simulink model "Test_per_emg"  (R2023b)
settings: Solver=VariableStepAuto  StartTime=0.0  StopTime=inf  RelTol=1e-3
undefined symbols (not defined in the file or in its folder): deg, m, s, t1, t2
libraries: qbmove_library x9, dspstat3 x2, CP_library x1, QB_pacer_lib x1
settings Model: Creator=ilari  LastModifiedBy=ilari

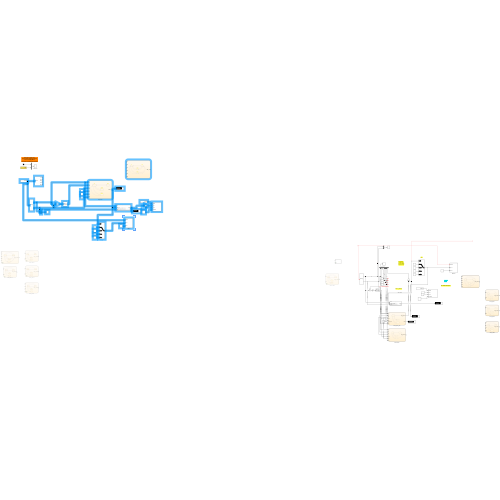
[thumbnail: Simulink's stored preview of the top-level diagram]
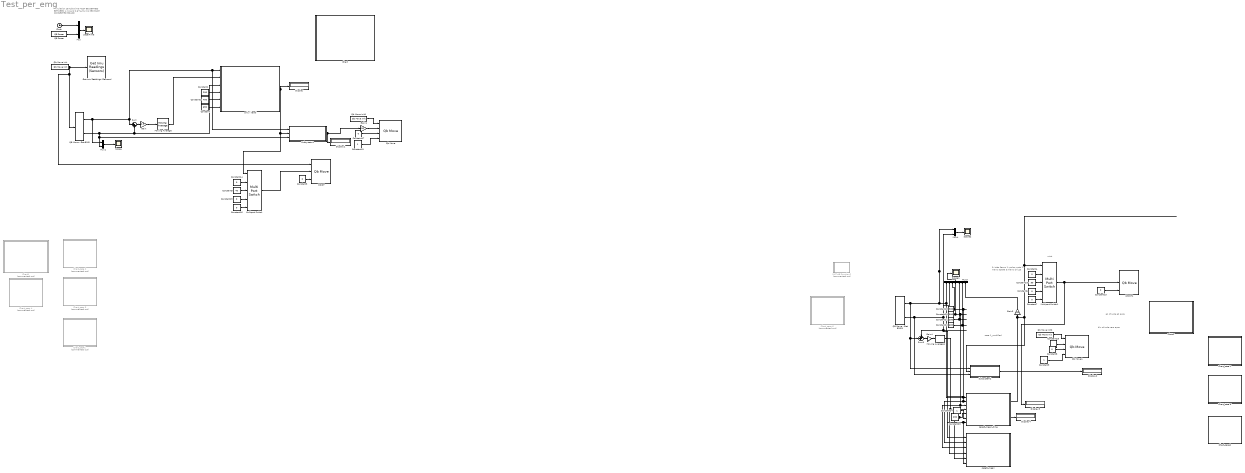
== system Test_per_emg ==
  note: Simulation sample time
      | MUST BE DEFINED BETWEEN
      | 1 ms and 0.6*N_IMU ms
      | PER EACH CONNECTED BOARD
  note: 0: tutto fermo
      | 1: polso ruota
      | 2: mano aperta
      | 3:mano chiusa
  note: wrist
  note: e1 chiude
      | e2 apre
  note: blu chiude nero apre
  note: case 1_modified
  Chart : Stateflow chart  TreatAsAtomicUnit=on
  Chart1 : Stateflow chart  Commented=on  TreatAsAtomicUnit=on
      settings: PortSchema="{\"entries\":[{\"content\":{\"sides\":[{\"content\":{\"connectorIds\":[\"In1\",\"In2\",\"In4\",\"In5\",\"In6\",\"In3\"]},\"type\":\"ConnectorPlacement.EquallySpacedRectSide\",\"uuid\":\"bb964aad-0f33-4b15-8f2f-07cc57dca142\"},{\"content\":{\"connectorIds\":[\"Out1\"],\"side\":\"RIGHT\"},\"type\":\"ConnectorPlacement.EquallySpacedRectSide\",\"uuid\":\"3d1bf315-7cf4-4964-aaea-501116c51cbb\"},{\"content\":{\"side\":\"TOP\"},\"type\":\"ConnectorPlacement.EquallySpacedRectSide\",\"uuid\":\"a0d71c19-2788-4f48-aff8-ceef882696bc\"}]},\"type\":\"ConnectorPlacement.EquallySpacedConnector\",\"uuid\":\"2eca7b29-df2d-4887-b2a9-df7a5d1fb129\"}],\"packageUris\":[\"http://schema.mathworks.com/mf0/Connector/R2020b\"],\"version\":\"1.0\"}"
  Chart2 : Stateflow chart  TreatAsAtomicUnit=on
      settings: PortSchema="{\"entries\":[{\"content\":{\"sides\":[{\"content\":{\"connectorIds\":[\"In1\",\"In2\",\"In4\",\"In5\",\"In6\",\"In3\"]},\"type\":\"ConnectorPlacement.EquallySpacedRectSide\",\"uuid\":\"bb964aad-0f33-4b15-8f2f-07cc57dca142\"},{\"content\":{\"connectorIds\":[\"Out1\"],\"side\":\"RIGHT\"},\"type\":\"ConnectorPlacement.EquallySpacedRectSide\",\"uuid\":\"3d1bf315-7cf4-4964-aaea-501116c51cbb\"},{\"content\":{\"side\":\"TOP\"},\"type\":\"ConnectorPlacement.EquallySpacedRectSide\",\"uuid\":\"a0d71c19-2788-4f48-aff8-ceef882696bc\"}]},\"type\":\"ConnectorPlacement.EquallySpacedConnector\",\"uuid\":\"2eca7b29-df2d-4887-b2a9-df7a5d1fb129\"}],\"packageUris\":[\"http://schema.mathworks.com/mf0/Connector/R2020b\"],\"version\":\"1.0\"}"
  Chart_case 1 : Stateflow chart  TreatAsAtomicUnit=on
  Chart_case 2 : Stateflow chart  Commented=on  TreatAsAtomicUnit=on
  Chart_case 3 : Stateflow chart  Commented=on  TreatAsAtomicUnit=on
  Chart_case 4 : Stateflow chart  Commented=on  TreatAsAtomicUnit=on
  Chart_case 5 : Stateflow chart  TreatAsAtomicUnit=on
  Chart_case 6 : Stateflow chart  Commented=on  TreatAsAtomicUnit=on
  Chart_case1 : Stateflow chart  Commented=on  TreatAsAtomicUnit=on
  Chart_case2 : Stateflow chart  TreatAsAtomicUnit=on
  Clock : Clock
  Constant : Constant  Value=650
  Constant1 : Constant  Value=200
  Constant10 : Constant  Value=50
  Constant{3..4,6..8,13..17} (10 alike) : Constant  Value=0
  Constant18 : Constant  Value=300
  Constant19 : Constant
  Constant2 : Constant  Value=400
  Constant20 : Constant  Value=500
  Constant21 : Constant  Value=200
  Constant22 : Constant  Value=600
  Constant23 : Constant  Value=230
  Constant24 : Constant
  Constant25 : Constant  Value=10000
  Constant5 : Constant  Value=40
  Constant9 : Constant
  Display{,1..4} (5 alike) : Display
  Gain : Gain  Gain=0.5
  Gain1 : Gain  Gain=50
  Gain3 : Gain  Gain=100
  Gain4 : Gain  Gain=0.5
  Get Imu Readings (Sensors) : CP_library/Get Imu Readings (Sensors)  ID=2  N_IMU=1  DAISY_CHAINING=off  ACC_UNITY=m/(s^2)  GYRO_UNITY=deg/s  MAG_UNITY=uT
      settings: SourceProductName=Centro Piaggio Library
  MATLAB Function5 : MATLAB Function  Commented=on  TreatAsAtomicUnit=on
  Moving Average : dspstat3/Moving Average  Method=Sliding window  ForgettingFactorPort=off  SpecifyWindowLength=on  WindowLength=4  OverlapLength=3  AllowArbitraryInputLength=off  ForgettingFactor=0.9  SimulateUsing=Code generation
  Moving Average1 : dspstat3/Moving Average  Method=Sliding window  ForgettingFactorPort=off  SpecifyWindowLength=on  WindowLength=4  OverlapLength=3  AllowArbitraryInputLength=off  ForgettingFactor=0.9  SimulateUsing=Code generation
  Multiport Switch : MultiPortSwitch  DataPortOrder=Zero-based contiguous  Inputs=4  zeroidx=on  SaturateOnIntegerOverflow=off  InputSameDT=off
  Multiport Switch1 : MultiPortSwitch  DataPortOrder=Zero-based contiguous  Inputs=4  zeroidx=on  SaturateOnIntegerOverflow=off  InputSameDT=off
  Mux : Mux  Inputs=2
  Mux1 : Mux  Inputs=2
  Mux3 : Mux  Inputs=7
  Mux4 : Mux  Inputs=2
  QB Move - Get EMG : qbmove_library/QB Move - Get EMG  ID=2  DAISY_CHAINING=off
      settings: SourceProductName=Qb Move Library
  QB Move - Get EMG1 : qbmove_library/QB Move - Get EMG  ID=2  DAISY_CHAINING=off
      settings: SourceProductName=Qb Move Library
  QB Pacer : QB_pacer_lib/QB Pacer  simTimePerRealTime=1
      settings: SourceProductName=QB Pacer
  Qb Move : qbmove_library/Qb Move  ID=1  ACTIVE_COMM_DIRECTIONS=Tx  CONTROL_MODE=Prime Movers Positions  DAISY_CHAINING=off  MAX_ANG=0  SW_LIMIT=inf  OFFSET=0  ACTIVATE=off  WDT=0.0  UNIT=TICK
      settings: LibrarySourceBlock=qbmove_library/qbmove  SourceProductName=Qb Move Library
  Qb Move Init : qbmove_library/Qb Move Init  NUMBER_OF_COM='COM9'  BAUD_RATE_COM=2000000
      settings: SourceProductName=Qb Move Library
  Qb Move Init1 : qbmove_library/Qb Move Init  NUMBER_OF_COM='COM7'  BAUD_RATE_COM=2000000
      settings: SourceProductName=Qb Move Library
  Qb Move Init2 : qbmove_library/Qb Move Init  NUMBER_OF_COM='COM7'  BAUD_RATE_COM=2000000
      settings: SourceProductName=Qb Move Library
  Qb Move1 : qbmove_library/Qb Move  ID=1  ACTIVE_COMM_DIRECTIONS=Tx  CONTROL_MODE=Prime Movers Positions  DAISY_CHAINING=off  MAX_ANG=0  SW_LIMIT=inf  OFFSET=0  ACTIVATE=off  WDT=0.0  UNIT=TICK
      settings: LibrarySourceBlock=qbmove_library/qbmove  SourceProductName=Qb Move Library
  Scope : Scope
  Scope1 : Scope
  Scope2 : Scope
  Subsystem1 : Subsystem
  Subsystem2 : Subsystem
  Sum : Sum  Inputs=|++
  Sum3 : Sum  Inputs=++|
  WRIST : qbmove_library/Qb Move  ID=2  ACTIVE_COMM_DIRECTIONS=Tx  CONTROL_MODE=Prime Movers Positions  DAISY_CHAINING=off  MAX_ANG=0  SW_LIMIT=inf  OFFSET=0  ACTIVATE=on  WDT=0.0  UNIT=TICK
      settings: SourceProductName=Qb Move Library
  WRIST1 : qbmove_library/Qb Move  ID=2  ACTIVE_COMM_DIRECTIONS=Tx  CONTROL_MODE=Prime Movers Positions  DAISY_CHAINING=off  MAX_ANG=0  SW_LIMIT=inf  OFFSET=0  ACTIVATE=on  WDT=0.0  UNIT=TICK
      settings: SourceProductName=Qb Move Library
  case5_mean : Stateflow chart  TreatAsAtomicUnit=on
      settings: PortSchema="{\"entries\":[{\"content\":{\"sides\":[{\"content\":{\"connectorIds\":[\"In1\",\"In2\",\"In4\",\"In6\",\"In5\",\"In3\"]},\"type\":\"ConnectorPlacement.EquallySpacedRectSide\",\"uuid\":\"bb964aad-0f33-4b15-8f2f-07cc57dca142\"},{\"content\":{\"connectorIds\":[\"Out1\"],\"side\":\"RIGHT\"},\"type\":\"ConnectorPlacement.EquallySpacedRectSide\",\"uuid\":\"3d1bf315-7cf4-4964-aaea-501116c51cbb\"},{\"content\":{\"side\":\"TOP\"},\"type\":\"ConnectorPlacement.EquallySpacedRectSide\",\"uuid\":\"a0d71c19-2788-4f48-aff8-ceef882696bc\"}]},\"type\":\"ConnectorPlacement.EquallySpacedConnector\",\"uuid\":\"2eca7b29-df2d-4887-b2a9-df7a5d1fb129\"}],\"packageUris\":[\"http://schema.mathworks.com/mf0/Connector/R2020b\"],\"version\":\"1.0\"}"
  case5_mean_time : Stateflow chart  TreatAsAtomicUnit=on
      settings: PortSchema="{\"entries\":[{\"content\":{\"sides\":[{\"content\":{\"connectorIds\":[\"In1\",\"In2\",\"In4\",\"In5\",\"In6\",\"In7\",\"In3\"]},\"type\":\"ConnectorPlacement.EquallySpacedRectSide\",\"uuid\":\"bb964aad-0f33-4b15-8f2f-07cc57dca142\"},{\"content\":{\"connectorIds\":[\"Out1\",\"Out2\"],\"side\":\"RIGHT\"},\"type\":\"ConnectorPlacement.EquallySpacedRectSide\",\"uuid\":\"3d1bf315-7cf4-4964-aaea-501116c51cbb\"},{\"content\":{\"side\":\"TOP\"},\"type\":\"ConnectorPlacement.EquallySpacedRectSide\",\"uuid\":\"a0d71c19-2788-4f48-aff8-ceef882696bc\"}]},\"type\":\"ConnectorPlacement.EquallySpacedConnector\",\"uuid\":\"2eca7b29-df2d-4887-b2a9-df7a5d1fb129\"}],\"packageUris\":[\"http://schema.mathworks.com/mf0/Connector/R2020b\"],\"version\":\"1.0\"}"
  only I level : Stateflow chart  TreatAsAtomicUnit=on
  pacerTime : Scope
  wires:
  Mux/1 -> pacerTime/1
  Clock/1 -> Mux/1
  QB Pacer/1 -> Mux/2
  Qb Move Init/1 -> WRIST/1, QB Move - Get EMG/1, Get Imu Readings (Sensors)/1
  QB Move - Get EMG/1 -> Mux1/1, Sum/1, only I level/1(e1), Subsystem1/1(e1)  "e1"
  QB Move - Get EMG/2 -> Mux1/2, Subsystem1/3(e2), only I level/3(e2), Sum/2  "e2"
  Sum/1 -> Gain/1
  Gain/1 -> Moving Average/1
  only I level/1(state_var) -> Multiport Switch/1, Subsystem1/2(In2), Display/1
  Constant/1 -> only I level/6(th2)
  Constant1/1 -> only I level/4(tm)
  Moving Average/1 -> only I level/2(em)
  Mux1/1 -> Scope/1
  Constant2/1 -> only I level/5(th1)
  Constant17/1 -> Qb Move/3
  Constant19/1 -> Qb Move/4
  Qb Move Init1/1 -> Qb Move/1
  Constant3/1 -> WRIST/3
  Multiport Switch/1 -> WRIST/2
  Constant16/1 -> Multiport Switch/5
  Constant14/1 -> Multiport Switch/2
  Constant15/1 -> Multiport Switch/4
  Constant5/1 -> Multiport Switch/3
  Subsystem1/1(Out1) -> Gain1/1, Display1/1
  Gain1/1 -> Qb Move/2
  Gain3/1 -> Mux3/7
  Constant24/1 -> case5_mean_time/7(time_min)
  Constant9/1 -> Qb Move1/4
  Gain4/1 -> Moving Average1/1
  Multiport Switch1/1 -> WRIST1/2, Display3/1
  case5_mean_time/2(time) -> Display4/1
  Constant6/1 -> Multiport Switch1/4
  Constant23/1 -> case5_mean_time/6(tm), case5_mean/5(tm)
  Qb Move Init2/1 -> Qb Move1/1
  Constant21/1 -> Mux3/5  "t3"
  Subsystem2/1(Out1) -> Display2/1
  Constant18/1 -> case5_mean/2(t1), case5_mean_time/2(t1), Mux3/3  "t1"
  Constant22/1 -> Mux3/6  "t4"
  Constant13/1 -> WRIST1/3
  Sum3/1 -> Gain4/1
  Mux3/1 -> Scope1/1
  Constant7/1 -> Multiport Switch1/5
  Constant4/1 -> Multiport Switch1/2
  Constant8/1 -> Qb Move1/3
  QB Move - Get EMG1/1 -> Mux4/1, Mux3/1, case5_mean/1(e1), case5_mean_time/1(e1), Sum3/2, Subsystem2/1(e1)  "e1"
  QB Move - Get EMG1/2 -> case5_mean/3(e2), case5_mean_time/3(e2), Sum3/1, Mux3/2, Mux4/2, Subsystem2/3(e2)  "e2"
  case5_mean_time/1(emg_control) -> Subsystem2/2(In2), Multiport Switch1/1, Gain3/1  "emg_control"
  Constant20/1 -> case5_mean_time/4(t2), case5_mean/4(t2), Mux3/4  "t2"
  Mux4/1 -> Scope2/1
  Constant10/1 -> Multiport Switch1/3
  Moving Average1/1 -> case5_mean_time/5(em), case5_mean/6(em)  "em"
  ? -> WRIST1/1
  ? -> QB Move - Get EMG1/1
  Constant25/1 -> Qb Move1/2

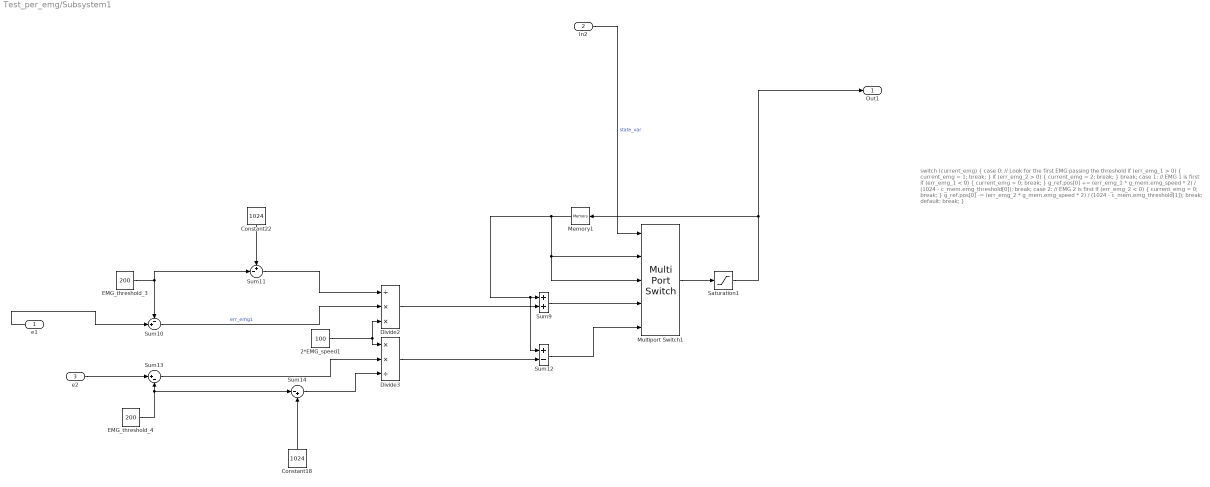
== system Test_per_emg/Subsystem1 ==
  note: switch (current_emg) {
      | case 0:
      | // Look for the first EMG passing the threshold
      | if (err_emg_1 > 0) {
      | current_emg = 1;
      | break;
      | }
      | if (err_emg_2 > 0) {
      | current_emg = 2;
      | break;
      | }
      | break;
      |
      | case 1:
      | // EMG 1 is first
      | if (err_emg_1 < 0) {
      | current_emg = 0;
      | break;
      | }
      | g_ref.pos[0] += (err_emg_1 * g_mem.emg_speed * 2) / (1024 - c_mem.emg_threshold[0]);
      | break;
      |
      | case 2:
      | // EMG 2 is first
      | if (err_emg_2 < 0) {
      | current_emg = 0;
      | break;
      | }
      | g_ref.pos[0] -= (err_emg_2 * g_mem.emg_speed * 2) / (1024 - c_mem.emg_threshold[1]);
      | break;
      |
      | default:
      | break;
      | }
  e1 : Inport
  In2 : Inport  Port=2
  e2 : Inport  Port=3
  2*EMG_speed1 : Constant  Value=100
  Constant18 : Constant  Value=1024
  Constant22 : Constant  Value=1024
  Divide2 : Product  Inputs=/**
  Divide3 : Product  Inputs=**/
  EMG_threshold_3 : Constant  Value=200
  EMG_threshold_4 : Constant  Value=200
  Memory1 : Memory
  Multiport Switch1 : MultiPortSwitch  DataPortOrder=Zero-based contiguous  Inputs=4  zeroidx=on  SaturateOnIntegerOverflow=off  InputSameDT=off
  Saturation1 : Saturate  UpperLimit=17500  LowerLimit=0
  Sum10 : Sum  Inputs=-+|
  Sum11 : Sum  Inputs=+-|
  Sum12 : Sum  Inputs=+-
  Sum13 : Sum  Inputs=|+-
  Sum14 : Sum  Inputs=|-+
  Sum9 : Sum
  Out1 : Outport
  wires:
  Multiport Switch1/1 -> Saturation1/1
  Memory1/1 -> Multiport Switch1/2, Multiport Switch1/3, Sum12/1, Sum9/1
  e1/1 -> Sum10/2
  Sum11/1 -> Divide2/1
  Sum9/1 -> Multiport Switch1/4
  Saturation1/1 -> Out1/1, Memory1/1
  Divide2/1 -> Sum9/2
  Divide3/1 -> Sum12/2
  Sum14/1 -> Divide3/3
  EMG_threshold_3/1 -> Sum11/2, Sum10/1
  EMG_threshold_4/1 -> Sum14/1, Sum13/2
  Constant18/1 -> Sum14/2
  2*EMG_speed1/1 -> Divide3/1, Divide2/3
  Sum13/1 -> Divide3/2
  e2/1 -> Sum13/1
  Sum12/1 -> Multiport Switch1/5
  Sum10/1 -> Divide2/2  "err_emg1"
  Constant22/1 -> Sum11/1
  In2/1 -> Multiport Switch1/1  "state_var"

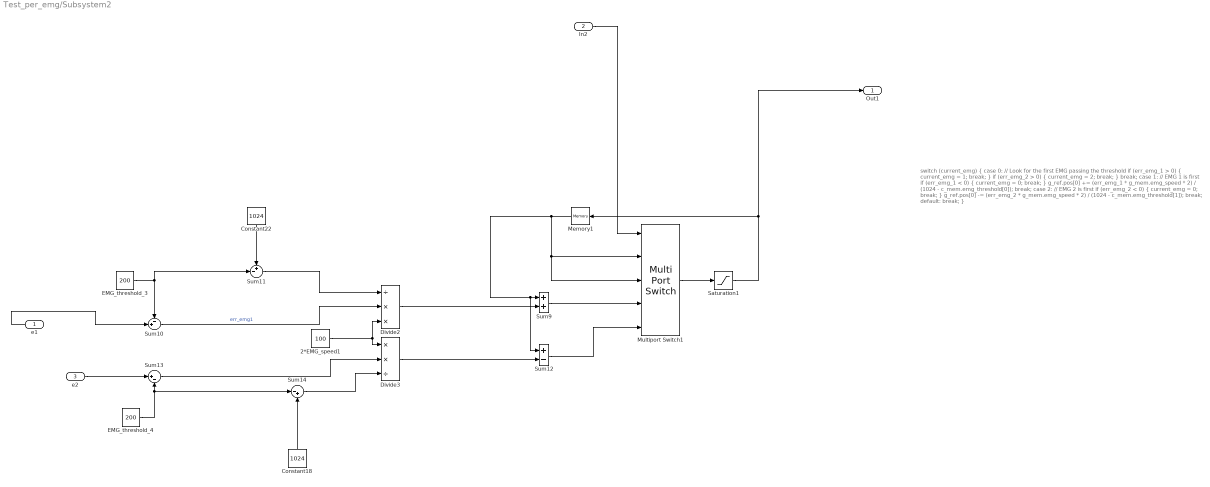
== system Test_per_emg/Subsystem2 ==
  note: switch (current_emg) {
      | case 0:
      | // Look for the first EMG passing the threshold
      | if (err_emg_1 > 0) {
      | current_emg = 1;
      | break;
      | }
      | if (err_emg_2 > 0) {
      | current_emg = 2;
      | break;
      | }
      | break;
      |
      | case 1:
      | // EMG 1 is first
      | if (err_emg_1 < 0) {
      | current_emg = 0;
      | break;
      | }
      | g_ref.pos[0] += (err_emg_1 * g_mem.emg_speed * 2) / (1024 - c_mem.emg_threshold[0]);
      | break;
      |
      | case 2:
      | // EMG 2 is first
      | if (err_emg_2 < 0) {
      | current_emg = 0;
      | break;
      | }
      | g_ref.pos[0] -= (err_emg_2 * g_mem.emg_speed * 2) / (1024 - c_mem.emg_threshold[1]);
      | break;
      |
      | default:
      | break;
      | }
  e1 : Inport
  In2 : Inport  Port=2
  e2 : Inport  Port=3
  2*EMG_speed1 : Constant  Value=100
  Constant18 : Constant  Value=1024
  Constant22 : Constant  Value=1024
  Divide2 : Product  Inputs=/**
  Divide3 : Product  Inputs=**/
  EMG_threshold_3 : Constant  Value=200
  EMG_threshold_4 : Constant  Value=200
  Memory1 : Memory
  Multiport Switch1 : MultiPortSwitch  DataPortOrder=Zero-based contiguous  Inputs=4  zeroidx=on  SaturateOnIntegerOverflow=off  InputSameDT=off
  Saturation1 : Saturate  UpperLimit=17500  LowerLimit=0
  Sum10 : Sum  Inputs=-+|
  Sum11 : Sum  Inputs=+-|
  Sum12 : Sum  Inputs=+-
  Sum13 : Sum  Inputs=|+-
  Sum14 : Sum  Inputs=|-+
  Sum9 : Sum
  Out1 : Outport
  wires:
  Multiport Switch1/1 -> Saturation1/1
  Memory1/1 -> Multiport Switch1/2, Multiport Switch1/3, Sum12/1, Sum9/1
  e1/1 -> Sum10/2
  Sum11/1 -> Divide2/1
  Sum9/1 -> Multiport Switch1/4
  Saturation1/1 -> Out1/1, Memory1/1
  Divide2/1 -> Sum9/2
  Divide3/1 -> Sum12/2
  Sum14/1 -> Divide3/3
  EMG_threshold_3/1 -> Sum11/2, Sum10/1
  EMG_threshold_4/1 -> Sum14/1, Sum13/2
  Constant18/1 -> Sum14/2
  2*EMG_speed1/1 -> Divide3/1, Divide2/3
  Sum13/1 -> Divide3/2
  e2/1 -> Sum13/1
  Sum12/1 -> Multiport Switch1/5
  Sum10/1 -> Divide2/2  "err_emg1"
  Constant22/1 -> Sum11/1
  In2/1 -> Multiport Switch1/1

== stateflow chart Test_per_emg/Chart_case 1 ==
  state State0
    entry: emg_control =0;
  state State1
    entry: emg_control=1;
  state State2
    entry: emg_control =2;
  state State3
    entry: emg_control=3;
  State1 -> State0 : [e2>t1 & e2<t2]
  (default) -> State0
  State0 -> State1 [order 2] : [e1>t1 & e1<t2]
  State0 -> State3 [order 3] : [e2>t2]
  State3 -> State0 : [e2<t2]
  State0 -> State2 [order 1] : [e1>t2]
  State2 -> State0 : [e1<t2]
  data: e1 input; e2 input; emg_control output; t2 parameter; t1 parameter

== stateflow chart Test_per_emg/Chart_case 5 ==
  state State0
    entry: emg_control =0;
  state State1
    entry: emg_control=1;
  state State2
    entry: emg_control =2;
  state State3
    entry: emg_control=3;
  State1 -> State0 : [e1>t1 & e1<t2]
  (default) -> State0
  State0 -> State1 [order 2] : [e2>t1 & e2<t2]
  State0 -> State3 [order 3] : [e2>t2]
  State3 -> State0 : [e2<t2]
  State0 -> State2 [order 1] : [e1>t2]
  State2 -> State0 : [e1<t2]
  data: e1 input; e2 input; emg_control output; t2 parameter; t1 parameter

== stateflow chart Test_per_emg/Chart_case 4 ==
  state State0
    entry: emg_control =0;
  state State1
    entry: emg_control=1;
  state State2
    entry: emg_control =2;
  state State3
    entry: emg_control=3;
  State1 -> State0 [order 2] : [e2>t1 & e2<t2]
  State1 -> State0 [order 1] : [e1>t1 & e1<t2]
  (default) -> State0
  State0 -> State1 [order 2] : [e1>t1 & e1<t2]
  State0 -> State1 [order 4] : [e2>t1 & e2<t2]
  State0 -> State3 [order 3] : [e2>t2]
  State3 -> State0 : [e2<t2]
  State0 -> State2 [order 1] : [e1>t2]
  State2 -> State0 : [e1<t2]
  data: e1 input; e2 input; emg_control output; t2 parameter; t1 parameter

== stateflow chart Test_per_emg/Chart1 ==
  state State0
    entry: emg_control =0;
  state State1
    entry: emg_control=1;
  state State2
    entry: emg_control =2;
  state State3
    entry: emg_control=3;
  State1 -> State0 [order 2] : [e1<t3]
  State1 -> State0 [order 1] : [e1<t3]
  (default) -> State0
  State0 -> State1 [order 2] : [e1>t1 & e1<t2]
  State0 -> State1 [order 4] : [e2>t1 & e2<t2]
  State1 -> State2 [order 4] : [e1>t4]
  State2 -> State1 [order 2] : [e1>t1 & e1<t2]
  State1 -> State3 [order 3] : [e2>t4]
  State3 -> State1 [order 2] : [e2>t1 & e2<t2]
  State0 -> State3 [order 3] : [e2>t2]
  State3 -> State0 [order 1] : [e2<t1]
  State0 -> State2 [order 1] : [e1>t2]
  State2 -> State0 [order 1] : [e1<t1]
  data: e1 input; t1 input; e2 input; t2 input; t3 input; t4 input; emg_control output

== stateflow chart Test_per_emg/Chart_case 2 ==
  state State0
    entry: emg_control =0;
  state State1
    entry: emg_control=1;
  state State2
    entry: emg_control =2;
  state State3
    entry: emg_control=3;
  State1 -> State0 : [e2>t1 & e2<t2]
  (default) -> State0
  State0 -> State1 [order 2] : [e1>t1 & e1<t2]
  State0 -> State3 [order 3] : [e2>t2]
  State3 -> State0 : [e2<t2]
  State0 -> State2 [order 1] : [e1>t2]
  State2 -> State0 : [e1<t2]
  data: e1 input; e2 input; emg_control output; t2 parameter; t1 parameter

== stateflow chart Test_per_emg/Chart_case 3 ==
  state State0
    entry: emg_control =0;
  state State1
    entry: emg_control=1;
  state State2
    entry: emg_control =2;
  state State3
    entry: emg_control=3;
  State1 -> State0 : [e1>t1 & e1<t2]
  (default) -> State0
  State0 -> State1 [order 2] : [e2>t1 & e2<t2]
  State0 -> State3 [order 3] : [e2>t2]
  State3 -> State0 : [e2<t2]
  State0 -> State2 [order 1] : [e1>t2]
  State2 -> State0 : [e1<t2]
  data: e1 input; e2 input; emg_control output; t2 parameter; t1 parameter

== stateflow chart Test_per_emg/Chart_case1 ==
  state State0
    entry: emg_control =0;
  state State1
    entry: emg_control=1;
  state State2
    entry: emg_control =2;
  state State3
    entry: emg_control=3;
  State1 -> State0 [order 2] : [e2>t2]
  State1 -> State0 [order 1] : [e1>t2]
  (default) -> State0
  State0 -> State1 [order 2] : [e1>t1 & e1<t2]
  State0 -> State1 [order 4] : [e2>t1 & e2<t2]
  State0 -> State3 [order 3] : [e2>t2]
  State3 -> State0 : [e2<t2]
  State0 -> State2 [order 1] : [e1>t2]
  State2 -> State0 : [e1<t2]
  data: e1 input; t1 input; t2 input; e2 input; emg_control output

== stateflow chart Test_per_emg/Chart_case 6 ==
  state State0
    entry: emg_control =0;
  state State1
    entry: emg_control=1;
  state State2
    entry: emg_control =2;
  state State3
    entry: emg_control=3;
  State1 -> State0 [order 2] : [e2>t1 & e2<t2]
  State1 -> State0 [order 1] : [e1>t1 & e1<t2]
  (default) -> State0
  State0 -> State1 [order 2] : [e1>t1 & e1<t2]
  State0 -> State1 [order 4] : [e2>t1 & e2<t2]
  State0 -> State3 [order 3] : [e2>t2]
  State3 -> State0 : [e2<t2]
  State0 -> State2 [order 1] : [e1>t2]
  State2 -> State0 : [e1<t2]
  data: e1 input; e2 input; emg_control output; t2 parameter; t1 parameter

== stateflow chart Test_per_emg/Chart_case2 ==
  state State0
    entry: emg_control =0;
  state State1
    entry: emg_control=1;
  state State2
    entry: emg_control =2;
  state State3
    entry: emg_control=3;
  State1 -> State0 [order 2] : [e2>t2]
  State1 -> State0 [order 1] : [e1>t2]
  (default) -> State0
  State0 -> State1 [order 2] : [e1>t1 & e1<t2]
  State0 -> State1 [order 4] : [e2>t1 & e2<t2]
  State0 -> State3 [order 3] : [e2>t2]
  State3 -> State0 : [e2<t2]
  State0 -> State2 [order 1] : [e1>t2]
  State2 -> State0 : [e1<t2]
  data: e1 input; t1 input; t2 input; e2 input; emg_control output

== matlab function Test_per_emg/MATLAB Function5 ==
  data: e1 input; e2 input
function  plot_emg(e1,e2)
figure(1)
hold on

yline(ax, 0.5, '--k', 'Linea di riferimento 1');
yline(ax, -0.5, '--k', 'Linea di riferimento 2');
plot (e1)
end

% persistent fig ax label_handle time
% 
% % Inizializza il grafico al primo ciclo
% if isempty(fig)
%     fig = figure;
%     ax = axes('Parent', fig);
%     hold(ax, 'on');
%     plot(ax, NaN, NaN, 'b', 'DisplayName', 'e1');
%     plot(ax, NaN, NaN, 'r', 'DisplayName', 'e2');
% 
%     % Aggiungi linee orizzontali di riferimento
%     yline(ax, 0.5, '--k', 'Linea di riferimento 1');
%     yline(ax, -0.5, '--k', 'Linea di riferimento 2');
% 
%     % Configura il grafico
%     xlabel(ax, 'Tempo (s)');
%     ylabel(ax, 'Valore');
%     title(ax, 'Grafico con etichetta dinamica e linee di riferimento');
%     legend(ax, 'show');
% 
%     time = 0;  % inizializza il tempo
% end
% 
% % Aggiorna il tempo a ogni chiamata (in Simulink questo viene aggiornato a ogni step)
% time = time + 0.1; % aggiorna il tempo, usando il passo di simulazione desiderato
% 
% % Plotta i dati aggiornati
% plot(ax, time, e1, 'bo');
% plot(ax, time, e2, 'ro');
% 
% % Crea o aggiorna l'etichetta dinamica
% if e1 > 0.7 && e2 > 0.7
%     label_text = 'Entrambi i segnali sopra la soglia 1';
% elseif e1 < -0.7 && e2 < -0.7
%     label_text = 'Entrambi i segnali sotto la soglia 2';
% else
%     label_text = 'Condizione neutrale';
% end
% 
% % Aggiorna o crea l'oggetto del testo
% if isempty(label_handle)
%     label_handle = text(time, max(e1, e2) + 0.1, label_text, ...
%         'FontSize', 10, 'FontWeight', 'bold', 'Color', 'm', 'Parent', ax);
% else
%     set(label_handle, 'Position', [time, max(e1, e2) + 0.1, 0], 'String', label_text);
% end
% 
% % Aggiorna gli assi per mantenere visibile l'ultimo valore
% xlim(ax, [max(0, time - 10), time + 1]); % visualizza solo gli ultimi 10 secondi
% 
% end

== stateflow chart Test_per_emg/case5_mean ==
  state State0
    entry: emg_control =0;
  state State1
    entry: emg_control=1;
  state State2
    entry: emg_control =2;
  state State3
    entry: emg_control=3;
  (default) -> State0
  State0 -> State1 [order 1] : [em>tm & e1<t2 & e2<t2]
  State1 -> State3 [order 2] : [em>tm & e1<t2 & e2>t2]
  State1 -> State0 [order 1] : [em<tm ]
  State1 -> State2 [order 3] : [em>tm & e1>t2 & e2<tm]
  State0 -> State3 [order 3] : [em>tm & e1<t2 & e2>t2]
  State3 -> State0 : [e2<t2]
  State2 -> State0 : [e1<t2 ]
  State0 -> State2 [order 2] : [em>tm & e1>t2 & e2<t2]
  data: e1 input; t1 input; e2 input; t2 input; tm input; emg_control output; em input

== stateflow chart Test_per_emg/case5_mean_time ==
  state State0
    entry: emg_control =0;
    entry: time =0;
    during: time = time +1;
    exit: time=0;
  state State1
    entry: emg_control=1;
  state State2
    entry: emg_control =2;
  state State3
    entry: emg_control=3;
  (default) -> State0
  State0 -> State1 [order 1] : [em>tm & e1<t2 & e2<t2 & time>time_min]
  State1 -> State0 : [em<tm & time>time_min]
  State0 -> State3 [order 3] : [em>tm & e1<t2 & e2>t1 & time>time_min]
  State3 -> State0 : [e2<t2 & time>time_min]
  State2 -> State0 : [e1<t2 & time>time_min]
  State0 -> State2 [order 2] : [em>tm & e1>t2 & e2<t2 & time>time_min]
  data: e1 input; t1 input; e2 input; t2 input; emg_control output; em input; tm input; time_min input; time output

== stateflow chart Test_per_emg/only I level ==
  note: rest
  note: polso on
  state state0
    entry: state_var = 0;
  state state1
    entry: state_var=1;
  note: mano chiusa
  state state2
    entry: state_var=2;
  note: mano aperta
  state state3
    entry: state_var=3;
  (default) -> state0
  state0 -> state1 [order 1] : [em>tm & e1<th1 & e2<th2]
  state1 -> state0 : [em<tm]
  state3 -> state0 : [em<tm & e2<th2]
  state0 -> state3 [order 3] : [em>tm & e2>th2]
  state0 -> state2 [order 2] : [em<tm & e1>th1]
  state2 -> state0 : [em<tm & e1<th1]
  data: e1 input; em input size=1; e2 input; tm input; th1 input; state_var output; th2 input

== stateflow chart Test_per_emg/Chart2 ==
  state State0
    entry: emg_control =0;
  state State1
    entry: emg_control=1;
  state State2
    entry: emg_control =2;
  state State3
    entry: emg_control=3;
  State1 -> State0 [order 2] : [e1<t3]
  State1 -> State0 [order 1] : [e1<t3]
  (default) -> State0
  State0 -> State1 [order 2] : [e1>t1 & e1<t2]
  State0 -> State1 [order 4] : [e2>t1 & e2<t2]
  State1 -> State2 [order 4] : [e1>t4]
  State2 -> State1 [order 2] : [e1>t1 & e1<t2]
  State1 -> State3 [order 3] : [e2>t4]
  State3 -> State1 [order 2] : [e2>t1 & e2<t2]
  State0 -> State3 [order 3] : [e2>t2]
  State3 -> State0 [order 1] : [e2<t1]
  State0 -> State2 [order 1] : [e1>t2]
  State2 -> State0 [order 1] : [e1<t1]
  data: e1 input; t1 input; e2 input; t2 input; t3 input; t4 input; emg_control output

== stateflow chart Test_per_emg/Chart ==
  note: rest
  note: polso on
  state state0
    entry: state_var = 0;
  state state1
    entry: state_var=1;
  note: mano chiusa
  state state2
    entry: state_var=2;
  note: mano aperta
  state state3
    entry: state_var=3;
  (default) -> state0
  state0 -> state1 [order 1] : [em>tm & e1<th1 & e2<th2]
  state1 -> state0 [order 1] : [em<tm]
  state1 -> state3 [order 2] : [em>tm & e2>th2]
  state3 -> state0 [order 2] : [em<tm & e2<th2]
  state3 -> state1 [order 1] : [em>tm & e2<th2]
  state0 -> state3 [order 3] : [em>tm & e2>th2]
  state0 -> state2 [order 2] : [em<tm & e1>th1]
  state2 -> state0 [order 2] : [em<tm & e1<th1]
  state2 -> state1 [order 1] : [em>tm &e1<th1]
  state1 -> state2 [order 3] : [em>tm & e1>th1 ]
  data: e1 input; em input size=1; e2 input; tm input; th1 input; state_var output; th2 input
